simulink model "dc_motor_with_encoder_control"  (R2024b)
settings: Solver=FixedStepDiscrete  StartTime=0.0  StopTime=inf  FixedStep=0.01  RelTol=1e-3  EnableMultiTasking=on
libraries: simulink x6, arduinolib x3, arduinosensorlib x1
settings Model: ExtModeTrigDuration=2  Creator=LENOVO  LastModifiedBy=LENOVO
settings SolverCC: AutoInsertRateTranBlk=on
settings OptimizationCC: EnhancedBackFolding=on  PassReuseOutputArgsAs=Individual arguments  ZeroExternalMemoryAtStartup=off  ZeroInternalMemoryAtStartup=off  MaxStackSize=64  OptimizeBlockOrder=speed  DifferentSizesBufferReuse=on  OptimizationCustomize=off  EfficientTunableParamExpr=on
settings DebuggingCC: ParameterTunabilityLossMsg=error
settings HardwareCC: ProdBitPerInt=16  ProdBitPerPointer=16  ProdBitPerSizeT=16  ProdBitPerPtrDiffT=16  ProdLargestAtomicFloat=None  ProdWordSize=8  ProdHWDeviceType=Atmel->AVR
settings SFSimCC: MATLABDynamicMemAlloc=off
settings RTWCC: Description=Embedded Coder  SystemTargetFile=ert.tlc  HardwareBoard=Arduino Uno  TemplateMakefile=ert_default_tmf  Toolchain=Arduino AVR  BuildConfiguration=Faster Runs
settings CodeAppCC: ForceParamTrailComments=on  IgnoreCustomStorageClasses=off  OperatorAnnotations=on  SimulinkDataObjDesc=on  SFDataObjDesc=on  InsertBlockDesc=on
settings ERTTargetCC: SupportContinuousTime=on  SupportVariableSizeSignals=on  ExtModeTransport=3  ExtModeStaticAlloc=on  ExtModeAutomaticAllocSize=off  ExtModeStaticAllocSize=250  ExtModeMexFile=ext_xcp  ExtModeIntrfLevel=Level2 - Open  InlinedParameterPlacement=Hierarchical

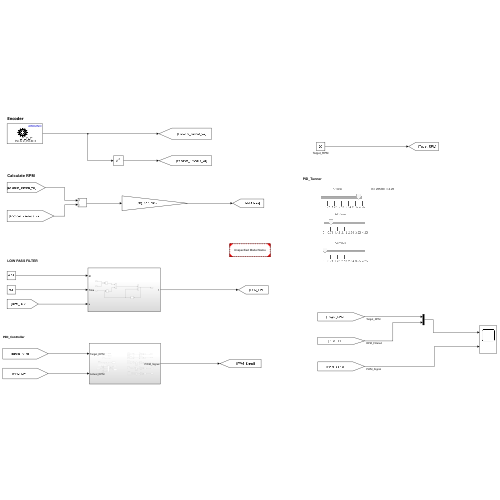
[thumbnail: Simulink's stored preview of the top-level diagram]
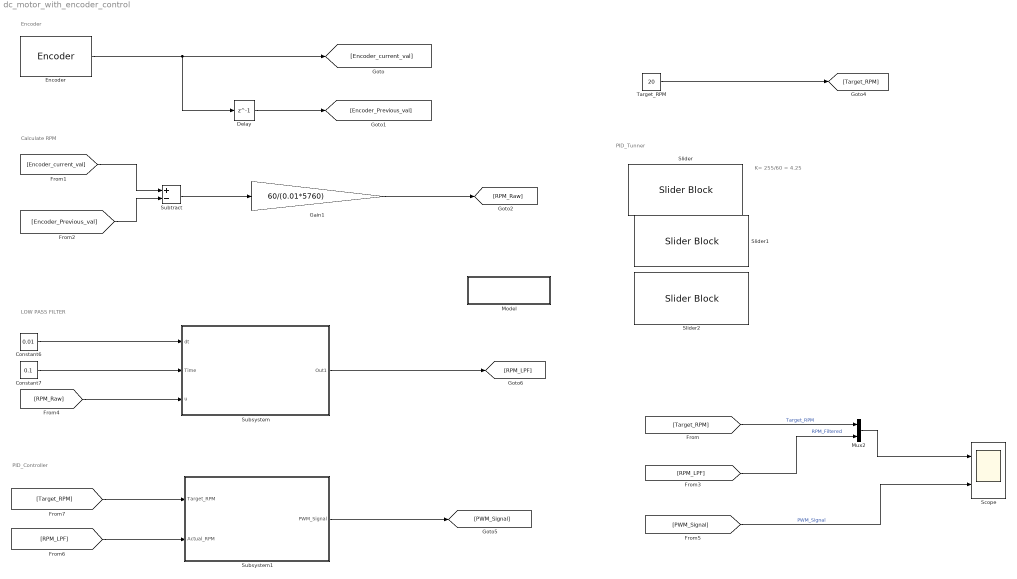
== system dc_motor_with_encoder_control ==
  note: K= 255/60 = 4.25
  note: PID_Tunner
  note: PID_Controller
  note: LOW PASS FILTER
  note: Encoder
  note: Calculate RPM
  Constant6 : Constant  Value=0.01  OutDataTypeStr=double
  Constant7 : Constant  Value=0.1  OutDataTypeStr=double
  Delay : Delay  DelayLength=1
  Encoder : arduinosensorlib/Encoder  InputA=2  InputB=3  Mode=No reset  SampleTime=0.01
      settings: SourceProductName=Sensors
  Gain1 : Gain  Gain=60/(0.01*5760)  OutDataTypeStr=double
  Model : ModelReference  SimulationMode=Normal
  Mux2 : Mux  Inputs=2
  Scope : Scope  NumInputPorts=2
  Slider : SliderBlock  ScaleMax=4.25
  Slider1 : SliderBlock  ScaleMax=4.25
  Slider2 : SliderBlock  ScaleMax=4.25
  Subsystem : Subsystem
  Subsystem1 : Subsystem
  Subtract : Sum  Inputs=+-  OutDataTypeStr=double
  Target_RPM : Constant  Value=20  OutDataTypeStr=double
  wires:
  Delay/1 -> [Encoder_Previous_val]
  Encoder/1 -> Delay/1, [Encoder_current_val]
  [Encoder_current_val] -> Subtract/1
  [Encoder_Previous_val] -> Subtract/2
  Subtract/1 -> Gain1/1
  Gain1/1 -> [RPM_Raw]
  Constant6/1 -> Subsystem/1(dt)
  Constant7/1 -> Subsystem/2(Time)
  [RPM_Raw] -> Subsystem/3(u)
  Subsystem/1(Out1) -> [RPM_LPF]
  [Target_RPM] -> Subsystem1/1(Target_RPM)
  Target_RPM/1 -> [Target_RPM]
  [Target_RPM] -> Mux2/1  "Target_RPM"
  [RPM_LPF] -> Mux2/2  "RPM_Filtered"
  [PWM_Signal] -> Scope/2  "PWM_Signal"
  Mux2/1 -> Scope/1
  Subsystem1/1(PWM_Signal) -> [PWM_Signal]
  [RPM_LPF] -> Subsystem1/2(Actual_RPM)

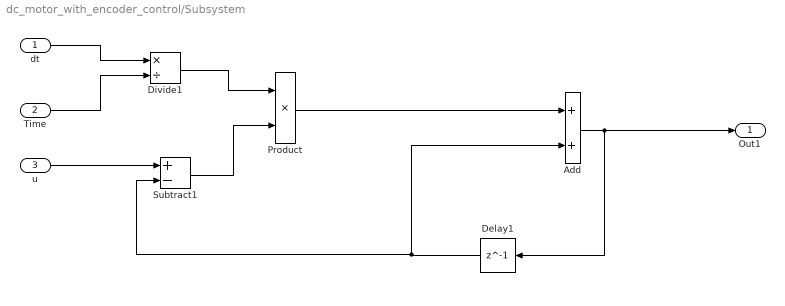
== system dc_motor_with_encoder_control/Subsystem ==
  dt : Inport  OutDataTypeStr=double
  Time : Inport  Port=2  OutDataTypeStr=double
  u : Inport  Port=3
  Add : Sum  OutDataTypeStr=double
  Delay1 : Delay  DelayLength=1
  Divide1 : Product  Inputs=*/
  Product : Product  OutDataTypeStr=double
  Subtract1 : Sum  Inputs=+-  OutDataTypeStr=double
  Out1 : Outport  OutDataTypeStr=double
  wires:
  Delay1/1 -> Subtract1/2, Add/2
  dt/1 -> Divide1/1
  Time/1 -> Divide1/2
  u/1 -> Subtract1/1
  Add/1 -> Out1/1, Delay1/1
  Product/1 -> Add/1
  Subtract1/1 -> Product/2
  Divide1/1 -> Product/1

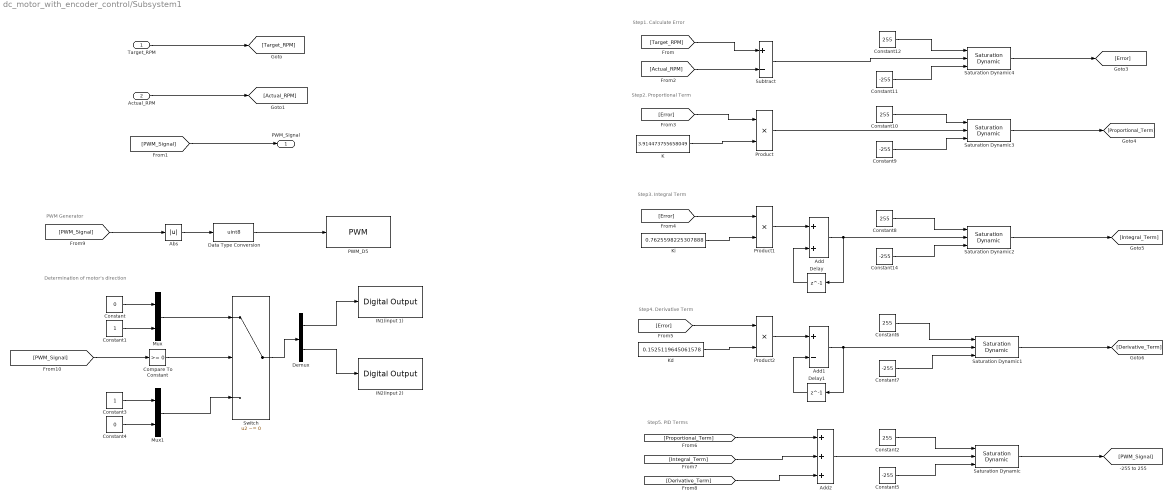
== system dc_motor_with_encoder_control/Subsystem1 ==
  note: Step1. Calculate Error
  note: Step5. PID Terms
  note: Step2. Proportional Term
  note: Step3. Integral Term
  note: Step4. Derivative Term
  note: PWM Generator
  note: Determination of motor's direction
  Target_RPM : Inport  OutDataTypeStr=double
  Actual_RPM : Inport  Port=2  OutDataTypeStr=double
  Abs : Abs  SaturateOnIntegerOverflow=off
  Add : Sum  OutDataTypeStr=int32
  Add1 : Sum  Inputs=+-  OutDataTypeStr=double
  Add2 : Sum  Inputs=+++  OutDataTypeStr=double
  Compare To Constant : simulink/Logic and Bit Operations/Compare To Constant  relop=>=  const=0  OutDataTypeStr=boolean
  Constant : Constant  Value=0  OutMin=0  OutMax=1  OutDataTypeStr=uint8
  Constant1 : Constant  OutMin=0  OutMax=1  OutDataTypeStr=uint8
  Constant{2,6,8,10,12} (5 alike) : Constant  Value=255  OutDataTypeStr=double
  Constant{5,7,9,11,14} (5 alike) : Constant  Value=-255  OutDataTypeStr=double
  Constant3 : Constant  OutMin=0  OutMax=1  OutDataTypeStr=uint8
  Constant4 : Constant  Value=0  OutMin=0  OutMax=1  OutDataTypeStr=uint8
  Data Type Conversion : DataTypeConversion  OutDataTypeStr=uint8  SaturateOnIntegerOverflow=off  RndMeth=Floor
  Delay : Delay  DelayLength=1
  Delay1 : Delay  DelayLength=1
  Demux : Demux  Outputs=2
  IN1(input 1) : arduinolib/Digital Output  pinNumber=9  Direction=output  blockPlatform=arduino
      settings: SourceProductName=Common
  IN2(input 2) : arduinolib/Digital Output  pinNumber=4  Direction=output  blockPlatform=arduino
      settings: SourceProductName=Common
  K : Constant  Value=3.914473755658049  OutDataTypeStr=double
  Kd : Constant  Value=0.1525119645061578  OutDataTypeStr=double
  Ki : Constant  Value=0.7625598225307888  OutDataTypeStr=double
  Mux : Mux  Inputs=2
  Mux1 : Mux  Inputs=2
  PWM_D5 : arduinolib/PWM  pinNumber=5  frequencyType=Default  desiredFrequency=490.2  achievableFrequency=490.2
      settings: SourceProductName=Common
  Product : Product  OutDataTypeStr=double
  Product1 : Product  OutDataTypeStr=double
  Product2 : Product  OutDataTypeStr=int32
  Saturation Dynamic{,1..4} (5 alike) : simulink/Discontinuities/Saturation Dynamic  OutMin=[]  OutMax=[]  OutDataTypeStr=double  OutDataType=fixdt(1, 16)  OutScaling=2^-10  DoSatur=off
  Subtract : Sum  Inputs=+-  OutDataTypeStr=double
  Switch : Switch  Criteria=u2 ~= 0  SaturateOnIntegerOverflow=off  InputSameDT=off
  PWM_Signal : Outport  OutDataTypeStr=double
  wires:
  Target_RPM/1 -> [Target_RPM]
  Actual_RPM/1 -> [Actual_RPM]
  [PWM_Signal] -> PWM_Signal/1
  [Target_RPM] -> Subtract/1
  [Actual_RPM] -> Subtract/2
  K/1 -> Product/2
  [Error] -> Product/1
  [Error] -> Product1/1
  Ki/1 -> Product1/2
  Product1/1 -> Add/1
  Add/1 -> Delay/1, Saturation Dynamic2/2
  Delay/1 -> Add/2
  Kd/1 -> Product2/2
  [Error] -> Product2/1
  Product2/1 -> Add1/1
  Add1/1 -> Saturation Dynamic1/2, Delay1/1
  Delay1/1 -> Add1/2
  [Integral_Term] -> Add2/2
  [Derivative_Term] -> Add2/3
  [Proportional_Term] -> Add2/1
  [PWM_Signal] -> Abs/1
  Abs/1 -> Data Type Conversion/1
  Data Type Conversion/1 -> PWM_D5/1
  Mux/1 -> Switch/1
  Constant4/1 -> Mux1/2
  Demux/2 -> IN2(input 2)/1
  Constant3/1 -> Mux1/1
  Constant/1 -> Mux/1
  Demux/1 -> IN1(input 1)/1
  Constant1/1 -> Mux/2
  Mux1/1 -> Switch/3
  Compare To Constant/1 -> Switch/2
  [PWM_Signal] -> Compare To Constant/1
  Switch/1 -> Demux/1
  Add2/1 -> Saturation Dynamic/2
  Constant2/1 -> Saturation Dynamic/1
  Constant5/1 -> Saturation Dynamic/3
  Saturation Dynamic/1 -> [PWM_Signal]
  Constant7/1 -> Saturation Dynamic1/3
  Saturation Dynamic1/1 -> [Derivative_Term]
  Constant6/1 -> Saturation Dynamic1/1
  Constant14/1 -> Saturation Dynamic2/3
  Saturation Dynamic2/1 -> [Integral_Term]
  Constant8/1 -> Saturation Dynamic2/1
  Constant9/1 -> Saturation Dynamic3/3
  Saturation Dynamic3/1 -> [Proportional_Term]
  Constant10/1 -> Saturation Dynamic3/1
  Product/1 -> Saturation Dynamic3/2
  Saturation Dynamic4/1 -> [Error]
  Subtract/1 -> Saturation Dynamic4/2
  Constant12/1 -> Saturation Dynamic4/1
  Constant11/1 -> Saturation Dynamic4/3
